simulink model "LB01B04"  (R2022b)
settings: Solver=ode45  StartTime=0.0  StopTime=20.0  MaxStep=0.01  RelTol=1e-3
settings Model: Creator=Andrey  LastModifiedBy=Andrey

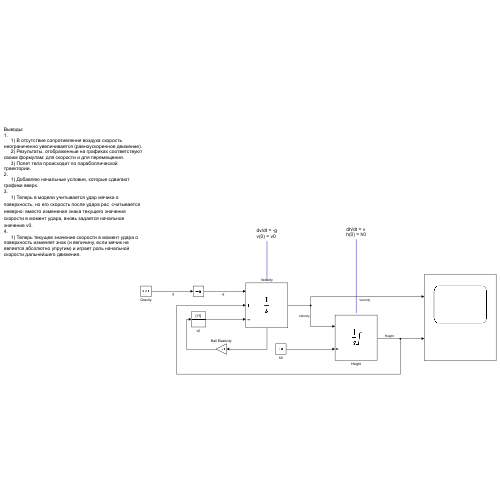
[thumbnail: Simulink's stored preview of the top-level diagram]
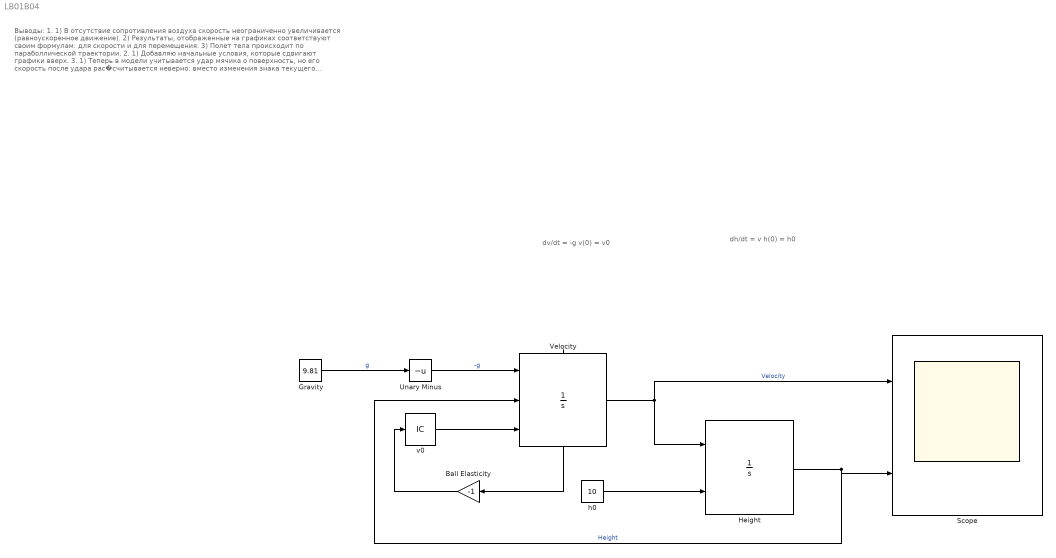
== system LB01B04 ==
  note: Выводы:
      | 1.
      | 1) В отсутствие сопротивления воздуха скорость неограниченно увеличивается (равноускоренное движение).
      | 2) Результаты, отображенные на графиках соответствуют своим формулам: для скорости и для перемещения.
      | 3) Полет тела происходит по параболлической траектории.
      | 2.
      | 1) Добавляю начальные условия, которые сдвигают графики вверх.
      | 3.
      | 1) Теперь в модели учитывается удар мячика о поверхность, но его скорость после удара рас�считывается неверно: вместо изменения знака текущего значения скорости в момент удара, вновь задается начальное значение v0.
      | 4.
      | 1) Теперь текущее значение скорости в момент удара о поверхность изменяет знак (и величину, если мячик не является абсолютно упругим) и играет роль начальной скорости дальнейшего движения.
  note: dh/dt = v
      | h(0) = h0
  note: dv/dt = -g
      | v(0) = v0
  Ball Elasticity : Gain  Gain=-1
  Gravity : Constant  Value=9.81
  Height : Integrator  InitialConditionSource=external  LimitOutput=on  LowerSaturationLimit=0
  Scope : Scope  NumInputPorts=2
  Unary Minus : UnaryMinus
  Velocity : Integrator  ExternalReset=falling  InitialConditionSource=external  InitialCondition=1  ShowStatePort=on
  h0 : Constant  Value=10
  v0 : InitialCondition  Value=15
  wires:
  Gravity/1 -> Unary Minus/1  "g"
  Unary Minus/1 -> Velocity/1  "-g"
  Velocity/1 -> Scope/1, Height/1  "Velocity"
  Height/1 -> Scope/2, Velocity/2  "Height"
  v0/1 -> Velocity/3
  h0/1 -> Height/2
  Velocity/State -> Ball Elasticity/1
  Ball Elasticity/1 -> v0/1
